simulink model "Backhoe_Arm_LS"  (R2013a)
settings: Solver=ode23t  StartTime=0.0  StopTime=30  MaxStep=0.01  RelTol=1e-3
PostLoadFcn:
  | warning off sm:compiler:state:UnsatisfiedDesiredTarget
  | warning off simscape:compiler:sli:init:SolverNotRecommended
  | warning off sm:sli:visualization:UnsupportedSimMode
  | warning off xPCTarget:sampleTime:sampleTimeInvariance
  | warning off sm:sli:setup:compile:LocalSolverNotSupported
model workspace (MAT data in the model file):
  cylinderGray = [0.6 0.6 0.6]
  darkOrange = [0.8 0.5 0]
  glassBlue = [0.2 0.2 1]
  gray = [0.3 0.3 0.3]
  orange = [0.8 0.65 0]
  pistonGray = [0.4 0.4 0.4]
  tireBlack = [0.1 0.1 0.1]
  wheelGray = [0.6 0.6 0.6]
  yellow = [0.8 0.8 0]
  rhoGlass = 2500
  rhoRubber = 1500
  rhoSteel = 7800
undefined symbols (not defined in the file or in its folder): BH_Param, sigbuilder_block, X, Y, Z
libraries: sm_lib x97, fl_lib x31, Backhoe_Lib x28, nesl_utility x21, sh_lib x9, xpclib x1
(part 2 of 4)

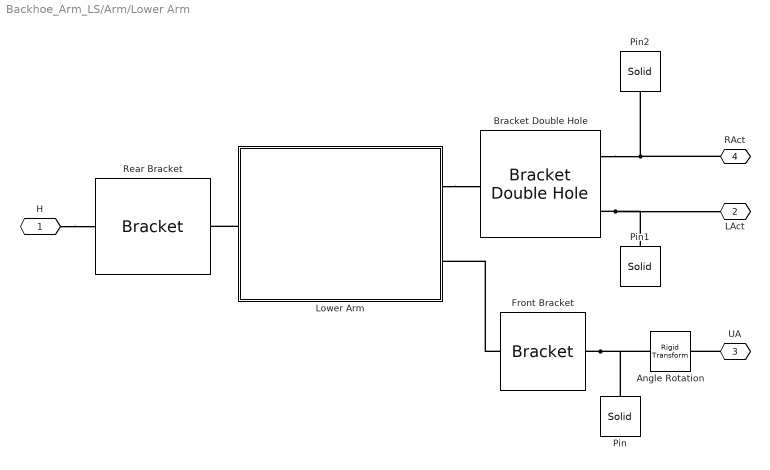
== system Backhoe_Arm_LS/Arm/Lower Arm  ==
  Angle Rotation : sm_lib/Frames and  Transforms/Rigid  Transform  TranslationMethod=None  TranslationLengthUnit=m  TranslationStandardAxis=+Z  TranslationStandardOffset=0  TranslationCartesianOffset=[0 0 0]  TranslationROffset=0  TranslationROffsetUnits=m  TranslationZOffset=0  TranslationZOffsetUnits=m  TranslationThetaOffset=0  TranslationThetaOffsetUnits=deg  RotationMethod=AlignedAxes  RotationAngleUnits=deg  RotationStandardAxis=+Z  RotationAngle=180  RotationArbitraryAxis=[0 0 1]  FollAlignAxisA=+Z  BaseAlignAxisA=+Z  FollAlignAxisB=+Y  BaseAlignAxisB=-Y  BlockFunction=simmechanics.library.frames_transforms.rigid_transform
  Bracket Double Hole : Backhoe_Lib/Bracket Double Hole  Hbracket=0.75  Wbracket=1.5  Tbracket=0.15  Dbracket=0.75  Hhole=0.5  Dhole=0.75  Rhole=0.075  Rfillet=0.375  Nc=25  bracketColor=orange  rho=rhoSteel
  Front Bracket : Backhoe_Lib/Bracket  Hbracket=0.65  Wbracket=0.5  Tbracket=0.225  Dbracket=0.45  Hhole=0.4  Rhole=0.075  circlePoints=25  bracketColor=darkOrange  rho=rhoSteel
  Lower Arm : Subsystem  mask(Lower Arm){Lbar=7, Wbar=0.8, Tbar=0.85, Lb=0.5, barFillet=0.1, numPoints=15, armColor=yellow, rho=rhoSteel}
      mask prompts: Lbar "Lbar [m]"; Wbar "Wbar [m]"; Tbar "Tbar [m]"; Lb "Lb [m]"; barFillet "Bar Fillet Radius [m]"; numPoints "Fillet Point Resolution"; armColor "Arm Color"; rho "Density [kg/m^3]"
      mask help:
      | Consists of the backhoe lower arm and three attachment brackets -- front, rear and upper
      |
      | Attachment Points are:
      | MA: Mounting Assembly attachment.
      | LH: Lower arm hydraulic actuator (piston Head).
      | UA: Upper arm attachment.
      | UC: Upper arm hydraulic actuator (Cylinder base).
      | All attachments are configured for Revolute joints.
      |
      | The length Lb corresponds to the lengths measured from the center of the bar to the center of the upper bracket.
      |
      | The front and rear brackets are automatically placed at the center of the end faces of the upper arm bar.
      |
      | Click on Help to view a schematic of the lower arm, its configurable dimension parameters and attachment points (in red).
      mask init:
      | barSection = [Tbar/2 Wbar/2;  ...
      |              -Tbar/2 Wbar/2;  ...
      |              -Tbar/2 -Wbar/2; ...
      |               Tbar/2 -Wbar/2];
      | barSection = Extr_Data_Round_Corners(barSection,1:4,barFillet,numPoints);
      mask Help: web('Backhoe_lowerarm.html');
      mask Display:
      | image(imread('Backhoe_Lowerarm_IMAGE.png'));
      | port_label('rconn',1,'RB');
      | port_label('lconn',2,'FB');;
      | port_label('lconn',1,'UB');
  Pin : sm_lib/Body Elements/Solid  InertiaType=CalculateFromGeometry  Mass=1  MassUnits=kg  CenterOfMass=[0 0 0]  CenterOfMassUnits=m  MomentsOfInertia=[1 1 1]  MomentsOfInertiaUnits=kg*m^2  ProductsOfInertia=[0 0 0]  ProductsOfInertiaUnits=kg*m^2  DensityBased=on  Density=rhoSteel  DensityUnits=kg/(m^3)  GraphicType=FromGeometry  MarkerShape=Sphere  MarkerSize=10  MarkerSizeUnits=m  GraphicVisPropType=SimpleVisualProperties  GraphicDiffuseColor=gray  GraphicSpecularColor=[0.5 0.5 0.5 1.0]  GraphicAmbientColor=[0.15 0.15 0.15 1.0]  GraphicEmissiveColor=[0.0 0.0 0.0 1.0]  GraphicShininess=75  GraphicOpacity=1.0  GeometryShape=Cylinder  RectangleSize=[1 1]  RectangleSizeUnits=m  BrickDimensions=[1 1 1]  BrickDimensionUnits=m  CylinderRadius=0.075  CylinderRadiusUnits=m  CylinderLength=0.8  CylinderLengthUnits=m  SphereRadius=1  SphereRadiusUnits=m  EllipsoidRadii=[1 1 1]  EllipsoidRadiiUnits=m  ExtrusionCrossSection=[1 1; -1 1; -1 -1; 1 -1]  ExtrusionCrossSectionUnits=m  ExtrusionLength=1  ExtrusionLengthUnits=m  PolygonNumSides=3  PolygonOuterRadius=1  PolygonOuterRadiusUnits=m  ExtGeomFileUnits=m  RevolutionCrossSection=[1 1; 1 -1; 2 -1; 2 1]  RevolutionCrossSectionUnits=m  RevolutionExtent=Full  RevolutionAngle=180  RevolutionAngleUnits=deg  BlockFunction=simmechanics.library.body_elements.solid
  Pin1 : sm_lib/Body Elements/Solid  InertiaType=CalculateFromGeometry  Mass=1  MassUnits=kg  CenterOfMass=[0 0 0]  CenterOfMassUnits=m  MomentsOfInertia=[1 1 1]  MomentsOfInertiaUnits=kg*m^2  ProductsOfInertia=[0 0 0]  ProductsOfInertiaUnits=kg*m^2  DensityBased=on  Density=rhoSteel  DensityUnits=kg/(m^3)  GraphicType=FromGeometry  MarkerShape=Sphere  MarkerSize=10  MarkerSizeUnits=m  GraphicVisPropType=SimpleVisualProperties  GraphicDiffuseColor=gray  GraphicSpecularColor=[0.5 0.5 0.5 1.0]  GraphicAmbientColor=[0.15 0.15 0.15 1.0]  GraphicEmissiveColor=[0.0 0.0 0.0 1.0]  GraphicShininess=75  GraphicOpacity=1.0  GeometryShape=Cylinder  RectangleSize=[1 1]  RectangleSizeUnits=m  BrickDimensions=[1 1 1]  BrickDimensionUnits=m  CylinderRadius=0.075  CylinderRadiusUnits=m  CylinderLength=0.8  CylinderLengthUnits=m  SphereRadius=1  SphereRadiusUnits=m  EllipsoidRadii=[1 1 1]  EllipsoidRadiiUnits=m  ExtrusionCrossSection=[1 1; -1 1; -1 -1; 1 -1]  ExtrusionCrossSectionUnits=m  ExtrusionLength=1  ExtrusionLengthUnits=m  PolygonNumSides=3  PolygonOuterRadius=1  PolygonOuterRadiusUnits=m  ExtGeomFileUnits=m  RevolutionCrossSection=[1 1; 1 -1; 2 -1; 2 1]  RevolutionCrossSectionUnits=m  RevolutionExtent=Full  RevolutionAngle=180  RevolutionAngleUnits=deg  BlockFunction=simmechanics.library.body_elements.solid
  Pin2 : sm_lib/Body Elements/Solid  InertiaType=CalculateFromGeometry  Mass=1  MassUnits=kg  CenterOfMass=[0 0 0]  CenterOfMassUnits=m  MomentsOfInertia=[1 1 1]  MomentsOfInertiaUnits=kg*m^2  ProductsOfInertia=[0 0 0]  ProductsOfInertiaUnits=kg*m^2  DensityBased=on  Density=rhoSteel  DensityUnits=kg/(m^3)  GraphicType=FromGeometry  MarkerShape=Sphere  MarkerSize=10  MarkerSizeUnits=m  GraphicVisPropType=SimpleVisualProperties  GraphicDiffuseColor=gray  GraphicSpecularColor=[0.5 0.5 0.5 1.0]  GraphicAmbientColor=[0.15 0.15 0.15 1.0]  GraphicEmissiveColor=[0.0 0.0 0.0 1.0]  GraphicShininess=75  GraphicOpacity=1.0  GeometryShape=Cylinder  RectangleSize=[1 1]  RectangleSizeUnits=m  BrickDimensions=[1 1 1]  BrickDimensionUnits=m  CylinderRadius=0.075  CylinderRadiusUnits=m  CylinderLength=0.8  CylinderLengthUnits=m  SphereRadius=1  SphereRadiusUnits=m  EllipsoidRadii=[1 1 1]  EllipsoidRadiiUnits=m  ExtrusionCrossSection=[1 1; -1 1; -1 -1; 1 -1]  ExtrusionCrossSectionUnits=m  ExtrusionLength=1  ExtrusionLengthUnits=m  PolygonNumSides=3  PolygonOuterRadius=1  PolygonOuterRadiusUnits=m  ExtGeomFileUnits=m  RevolutionCrossSection=[1 1; 1 -1; 2 -1; 2 1]  RevolutionCrossSectionUnits=m  RevolutionExtent=Full  RevolutionAngle=180  RevolutionAngleUnits=deg  BlockFunction=simmechanics.library.body_elements.solid
  Rear Bracket : Backhoe_Lib/Bracket  Hbracket=0.75  Wbracket=0.75  Tbracket=0.15  Dbracket=0.75  Hhole=0.5  Rhole=0.075  circlePoints=25  bracketColor=darkOrange  rho=rhoSteel
  H : PMIOPort  Port=1  Side=Left
  LAct : PMIOPort  Port=2  Side=Left
  UA : PMIOPort  Port=3  Side=Right
  RAct : PMIOPort  Port=4  Side=Right
  connections:
  H/RConn1 -- Rear Bracket/RConn1
  Lower Arm/RConn1 -- Rear Bracket/LConn1
  Front Bracket/RConn1 -- Pin/RConn1 -- Angle Rotation/LConn1
  Front Bracket/LConn1 -- Lower Arm/LConn2
  UA/RConn1 -- Angle Rotation/RConn1
  Lower Arm/LConn1 -- Bracket Double Hole/LConn1
  Bracket Double Hole/RConn2 -- LAct/RConn1 -- Pin1/RConn1
  Bracket Double Hole/RConn1 -- RAct/RConn1 -- Pin2/RConn1

== system Backhoe_Arm_LS/Arm/Measured ==
  Vector Concatenate : Concatenate  NumInputs=3
  Angles : Outport
  wires:
  [UA] -> Vector Concatenate/2
  Vector Concatenate/1 -> Angles/1
  [BuA] -> Vector Concatenate/1
  [LA] -> Vector Concatenate/3

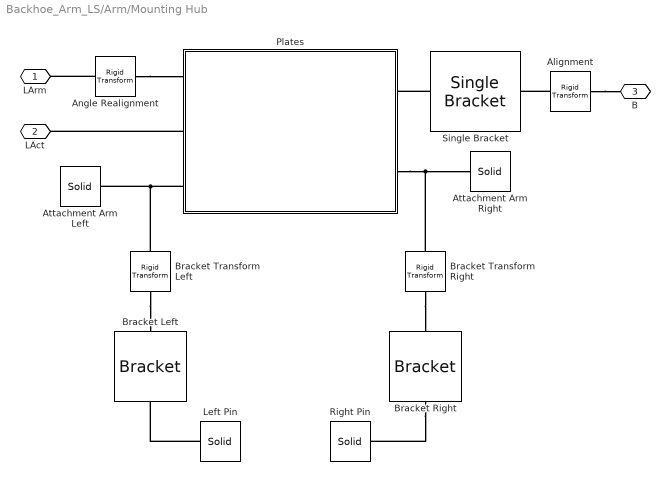
== system Backhoe_Arm_LS/Arm/Mounting Hub ==
  Alignment : sm_lib/Frames and  Transforms/Rigid  Transform  TranslationMethod=None  TranslationLengthUnit=m  TranslationStandardAxis=+Z  TranslationStandardOffset=0  TranslationCartesianOffset=[0 0 0]  TranslationROffset=0  TranslationROffsetUnits=m  TranslationZOffset=0  TranslationZOffsetUnits=m  TranslationThetaOffset=0  TranslationThetaOffsetUnits=deg  RotationMethod=StandardAxis  RotationAngleUnits=deg  RotationStandardAxis=+Y  RotationAngle=180  RotationArbitraryAxis=[0 0 1]  FollAlignAxisA=+X  BaseAlignAxisA=+X  FollAlignAxisB=+Y  BaseAlignAxisB=+Z  BlockFunction=simmechanics.library.frames_transforms.rigid_transform
  Angle Realignment : sm_lib/Frames and  Transforms/Rigid  Transform  TranslationMethod=None  TranslationLengthUnit=m  TranslationStandardAxis=+Z  TranslationStandardOffset=0.5  TranslationCartesianOffset=[ 0 0 0]  TranslationROffset=0  TranslationROffsetUnits=m  TranslationZOffset=0  TranslationZOffsetUnits=m  TranslationThetaOffset=0  TranslationThetaOffsetUnits=deg  RotationMethod=AlignedAxes  RotationAngleUnits=deg  RotationStandardAxis=-Z  RotationAngle=90  RotationArbitraryAxis=[0 0 1]  FollAlignAxisA=+Z  BaseAlignAxisA=+Z  FollAlignAxisB=+X  BaseAlignAxisB=-Y  BlockFunction=simmechanics.library.frames_transforms.rigid_transform
  Attachment Arm Left : sm_lib/Body Elements/Solid  InertiaType=CalculateFromGeometry  Mass=1  MassUnits=kg  CenterOfMass=[0 0 0]  CenterOfMassUnits=m  MomentsOfInertia=[1 1 1]  MomentsOfInertiaUnits=kg*m^2  ProductsOfInertia=[0 0 0]  ProductsOfInertiaUnits=kg*m^2  DensityBased=on  Density=rho  DensityUnits=kg/(m^3)  GraphicType=FromGeometry  MarkerShape=Sphere  MarkerSize=10  MarkerSizeUnits=m  GraphicVisPropType=SimpleVisualProperties  GraphicDiffuseColor=hubColor  GraphicSpecularColor=[0.5 0.5 0.5 1.0]  GraphicAmbientColor=[0.15 0.15 0.15 1.0]  GraphicEmissiveColor=[0.0 0.0 0.0 1.0]  GraphicShininess=75  GraphicOpacity=1.0  GeometryShape=Brick  RectangleSize=[1 1]  RectangleSizeUnits=m  BrickDimensions=[Warm Tarm (Larm-Warm)]  BrickDimensionUnits=m  CylinderRadius=1  CylinderRadiusUnits=m  CylinderLength=1  CylinderLengthUnits=m  SphereRadius=1  SphereRadiusUnits=m  EllipsoidRadii=[1 1 1]  EllipsoidRadiiUnits=m  ExtrusionCrossSection=plateSection  ExtrusionCrossSectionUnits=m  ExtrusionLength=Tplate  ExtrusionLengthUnits=m  PolygonNumSides=3  PolygonOuterRadius=1  PolygonOuterRadiusUnits=m  ExtGeomFileUnits=m  RevolutionCrossSection=[1 1; 1 -1; 2 -1; 2 1]  RevolutionCrossSectionUnits=m  RevolutionExtent=Full  RevolutionAngle=180  RevolutionAngleUnits=deg  BlockFunction=simmechanics.library.body_elements.solid
  Attachment Arm Right : sm_lib/Body Elements/Solid  InertiaType=CalculateFromGeometry  Mass=1  MassUnits=kg  CenterOfMass=[0 0 0]  CenterOfMassUnits=m  MomentsOfInertia=[1 1 1]  MomentsOfInertiaUnits=kg*m^2  ProductsOfInertia=[0 0 0]  ProductsOfInertiaUnits=kg*m^2  DensityBased=on  Density=rho  DensityUnits=kg/(m^3)  GraphicType=FromGeometry  MarkerShape=Sphere  MarkerSize=10  MarkerSizeUnits=m  GraphicVisPropType=SimpleVisualProperties  GraphicDiffuseColor=hubColor  GraphicSpecularColor=[0.5 0.5 0.5 1.0]  GraphicAmbientColor=[0.15 0.15 0.15 1.0]  GraphicEmissiveColor=[0.0 0.0 0.0 1.0]  GraphicShininess=75  GraphicOpacity=1.0  GeometryShape=Brick  RectangleSize=[1 1]  RectangleSizeUnits=m  BrickDimensions=[Warm Tarm (Larm-Warm)]  BrickDimensionUnits=m  CylinderRadius=1  CylinderRadiusUnits=m  CylinderLength=1  CylinderLengthUnits=m  SphereRadius=1  SphereRadiusUnits=m  EllipsoidRadii=[1 1 1]  EllipsoidRadiiUnits=m  ExtrusionCrossSection=plateSection  ExtrusionCrossSectionUnits=m  ExtrusionLength=Tplate  ExtrusionLengthUnits=m  PolygonNumSides=3  PolygonOuterRadius=1  PolygonOuterRadiusUnits=m  ExtGeomFileUnits=m  RevolutionCrossSection=[1 1; 1 -1; 2 -1; 2 1]  RevolutionCrossSectionUnits=m  RevolutionExtent=Full  RevolutionAngle=180  RevolutionAngleUnits=deg  BlockFunction=simmechanics.library.body_elements.solid
  Bracket Transform Left : sm_lib/Frames and  Transforms/Rigid  Transform  TranslationMethod=StandardAxis  TranslationLengthUnit=m  TranslationStandardAxis=+Z  TranslationStandardOffset=(Larm-Warm)/2  TranslationCartesianOffset=[0 0 0]  TranslationROffset=0  TranslationROffsetUnits=m  TranslationZOffset=0  TranslationZOffsetUnits=m  TranslationThetaOffset=0  TranslationThetaOffsetUnits=deg  RotationMethod=AlignedAxes  RotationAngleUnits=deg  RotationStandardAxis=+Y  RotationAngle=180  RotationArbitraryAxis=[0 0 1]  FollAlignAxisA=+Z  BaseAlignAxisA=+Z  FollAlignAxisB=+X  BaseAlignAxisB=+X  BlockFunction=simmechanics.library.frames_transforms.rigid_transform
  Bracket Transform Right : sm_lib/Frames and  Transforms/Rigid  Transform  TranslationMethod=StandardAxis  TranslationLengthUnit=m  TranslationStandardAxis=-Z  TranslationStandardOffset=(Larm-Warm)/2  TranslationCartesianOffset=[0 0 0]  TranslationROffset=0  TranslationROffsetUnits=m  TranslationZOffset=0  TranslationZOffsetUnits=m  TranslationThetaOffset=0  TranslationThetaOffsetUnits=deg  RotationMethod=AlignedAxes  RotationAngleUnits=deg  RotationStandardAxis=+Y  RotationAngle=180  RotationArbitraryAxis=[0 0 1]  FollAlignAxisA=+Z  BaseAlignAxisA=-Z  FollAlignAxisB=+Y  BaseAlignAxisB=+Y  BlockFunction=simmechanics.library.frames_transforms.rigid_transform
  Bracket Left : Backhoe_Lib/Bracket  Hbracket=Warm  Wbracket=Warm  Tbracket=Tab  Dbracket=Tarm  Hhole=Warm/2  Rhole=RH3  circlePoints=25  bracketColor=hubColor  rho=rho
  Bracket Right : Backhoe_Lib/Bracket  Hbracket=Warm  Wbracket=Warm  Tbracket=Tab  Dbracket=Tarm  Hhole=Warm/2  Rhole=RH3  circlePoints=25  bracketColor=hubColor  rho=rho
  Left Pin : sm_lib/Body Elements/Solid  InertiaType=CalculateFromGeometry  Mass=1  MassUnits=kg  CenterOfMass=[0 0 0]  CenterOfMassUnits=m  MomentsOfInertia=[1 1 1]  MomentsOfInertiaUnits=kg*m^2  ProductsOfInertia=[0 0 0]  ProductsOfInertiaUnits=kg*m^2  DensityBased=on  Density=rhoSteel  DensityUnits=kg/(m^3)  GraphicType=FromGeometry  MarkerShape=Sphere  MarkerSize=10  MarkerSizeUnits=m  GraphicVisPropType=SimpleVisualProperties  GraphicDiffuseColor=gray  GraphicSpecularColor=[0.5 0.5 0.5 1.0]  GraphicAmbientColor=[0.15 0.15 0.15 1.0]  GraphicEmissiveColor=[0.0 0.0 0.0 1.0]  GraphicShininess=75  GraphicOpacity=1.0  GeometryShape=Cylinder  RectangleSize=[1 1]  RectangleSizeUnits=m  BrickDimensions=[3 0.5 0.5]  BrickDimensionUnits=m  CylinderRadius=RH3  CylinderRadiusUnits=m  CylinderLength=Tarm*1.2  CylinderLengthUnits=m  SphereRadius=1  SphereRadiusUnits=m  EllipsoidRadii=[1 1 1]  EllipsoidRadiiUnits=m  ExtrusionCrossSection=[1 1; -1 1; -1 -1; 1 -1]  ExtrusionCrossSectionUnits=m  ExtrusionLength=1  ExtrusionLengthUnits=m  PolygonNumSides=3  PolygonOuterRadius=1  PolygonOuterRadiusUnits=m  ExtGeomFileUnits=m  RevolutionCrossSection=[1 1; 1 -1; 2 -1; 2 1]  RevolutionCrossSectionUnits=m  RevolutionExtent=Full  RevolutionAngle=180  RevolutionAngleUnits=deg  BlockFunction=simmechanics.library.body_elements.solid
  Plates : Subsystem
      mask Display:
      | image(imread('Backhoe_Mountingplates_IMAGE.png'));
      | port_label('lconn',1,'LA');
      | port_label('lconn',2,'LC');
      | port_label('lconn',3,'AAL');
      | port_label('rconn',1,'B');
      | port_label('rconn',2,'AAR');
  Right Pin : sm_lib/Body Elements/Solid  InertiaType=CalculateFromGeometry  Mass=1  MassUnits=kg  CenterOfMass=[0 0 0]  CenterOfMassUnits=m  MomentsOfInertia=[1 1 1]  MomentsOfInertiaUnits=kg*m^2  ProductsOfInertia=[0 0 0]  ProductsOfInertiaUnits=kg*m^2  DensityBased=on  Density=rhoSteel  DensityUnits=kg/(m^3)  GraphicType=FromGeometry  MarkerShape=Sphere  MarkerSize=10  MarkerSizeUnits=m  GraphicVisPropType=SimpleVisualProperties  GraphicDiffuseColor=gray  GraphicSpecularColor=[0.5 0.5 0.5 1.0]  GraphicAmbientColor=[0.15 0.15 0.15 1.0]  GraphicEmissiveColor=[0.0 0.0 0.0 1.0]  GraphicShininess=75  GraphicOpacity=1.0  GeometryShape=Cylinder  RectangleSize=[1 1]  RectangleSizeUnits=m  BrickDimensions=[3 0.5 0.5]  BrickDimensionUnits=m  CylinderRadius=RH3  CylinderRadiusUnits=m  CylinderLength=Tarm*1.2  CylinderLengthUnits=m  SphereRadius=1  SphereRadiusUnits=m  EllipsoidRadii=[1 1 1]  EllipsoidRadiiUnits=m  ExtrusionCrossSection=[1 1; -1 1; -1 -1; 1 -1]  ExtrusionCrossSectionUnits=m  ExtrusionLength=1  ExtrusionLengthUnits=m  PolygonNumSides=3  PolygonOuterRadius=1  PolygonOuterRadiusUnits=m  ExtGeomFileUnits=m  RevolutionCrossSection=[1 1; 1 -1; 2 -1; 2 1]  RevolutionCrossSectionUnits=m  RevolutionExtent=Full  RevolutionAngle=180  RevolutionAngleUnits=deg  BlockFunction=simmechanics.library.body_elements.solid
  Single Bracket : Backhoe_Lib/Single Bracket  Hbracket=Lbracket  Wbracket=Dplates-Tplate  Tbracket=Hright  Hhole=Hhole  Rhole=Rhole  Nc=25  bracketColor=orange  rho=rho
  LArm : PMIOPort  Port=1  Side=Right
  LAct : PMIOPort  Port=2  Side=Right
  B : PMIOPort  Port=3  Side=Left
  connections:
  Bracket Transform Right/RConn1 -- Bracket Right/LConn1
  Bracket Right/RConn1 -- Right Pin/RConn1
  Bracket Transform Right/LConn1 -- Plates/RConn2 -- Attachment Arm Right/RConn1
  Bracket Transform Left/RConn1 -- Bracket Left/LConn1
  Left Pin/RConn1 -- Bracket Left/RConn1
  Bracket Transform Left/LConn1 -- Plates/LConn3 -- Attachment Arm Left/RConn1
  Single Bracket/LConn1 -- Plates/RConn1
  Plates/LConn2 -- LAct/RConn1
  Alignment/LConn1 -- B/RConn1
  Alignment/RConn1 -- Single Bracket/RConn1
  Angle Realignment/LConn1 -- Plates/LConn1
  Angle Realignment/RConn1 -- LArm/RConn1

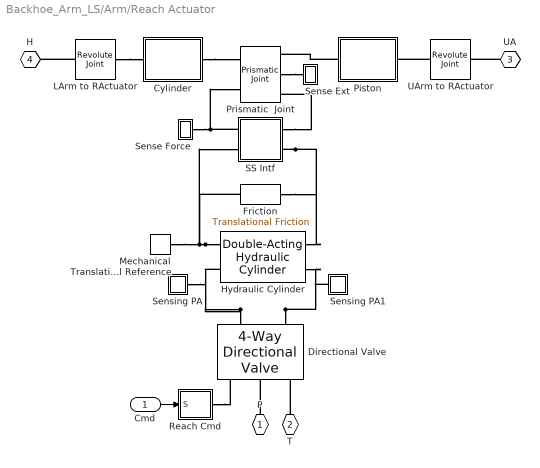
== system Backhoe_Arm_LS/Arm/Reach Actuator ==
  Cmd : Inport
  Cylinder : Subsystem
  Directional Valve : sh_lib/Valves/Directional Valves/4-Way Directional Valve  Tag=Factory Generic  mdl_type=1  area_max=hydr_valve_max_area mm^2  opening_max=hydr_valve_max_opening m  opening_tab="[  -0.002 0 0.005 0.015 ] m"  area_tab="[  1e-12 4e-12 1e-05 1.02e-05 ] m^2"  pressure_tab="[  -5e+06 -2e+06 2e+06 5e+06 ] Pa"  flow_rate_tab="[  -1e-12 -6e-14 6e+12 1e+11 ; -8e-08 -4e-08 4e+06 8e+06 ; -0.0025 -0.00103 0.001 0.0024 ; -0.00258 -0.001032 0.00106 0.00247 ; ] m^3/s"  interp_method=1  extrap_method=1  C_d=0.7  x_0_P_A=0 m  x_0_P_B=0 m  x_0_A_T=0 m  x_0_B_T=0 m  Re_cr=12  A_leak=1e-12 m^2  LocalVarLogging=[]
  Friction : fl_lib/Mechanical/Translational Elements/Translational Friction  brkwy_frc=friction_breakaway N  Col_frc=friction_coulomb N  visc_coef=friction_viscous N/(m/s)  trans_coef=10 s/m  vel_thr=1e-4 m/s  f_Log=off  v_Log=off  LocalVarNames=|f|v  LocalVarDescs=|f|v  LocalVarLogging=[0 0]
  Hydraulic Cylinder : sh_lib/Hydraulic Cylinders/Double-Acting Hydraulic Cylinder  Tag=Factory Generic  area_A=hydr_area m^2  area_B=hydr_area m^2  stroke=hydr_stroke m  init_pos=hydr_x0 m  dead_vol_A=hydr_deadvol m^3  dead_vol_B=hydr_deadvol m^3  init_pressure_A=hydr_PA0 Pa  init_pressure_B=hydr_PB0 Pa  k_sh=1.4  stiff=1e+06 N/m  D=150 N/(m/s)  or=2  LocalVarLogging=[]
  LArm to RActuator : sm_lib/Joints/Revolute Joint  SenseConstraintForceX=off  SenseConstraintForceY=off  SenseConstraintForceZ=off  SenseConstraintTorqueX=off  SenseConstraintTorqueY=off  SenseConstraintTorqueZ=off  ConstraintWrenchDir=FollowerOnBase  ConstraintWrenchFrame=BaseFrame  EquilibriumPosition=0  EquilibriumPositionUnits=deg  SpringStiffness=0  SpringStiffnessUnits=N*m/deg  DampingCoefficient=0  DampingCoefficientUnits=N*m/(deg/s)  ActuationMode=NoActuation  SensePosition=off  SenseVelocity=off  SenseAcceleration=off  SenseTorqueForce=off  PositionTargetValue=90  PositionTargetValueUnits=deg  PositionTargetSpecify=on  PositionTargetPriority=Low  VelocityTargetValue=0  VelocityTargetValueUnits=deg/s  VelocityTargetSpecify=off  VelocityTargetPriority=High  BlockFunction=simmechanics.library.joints.revolute_joint
  Mechanical Translational Reference : fl_lib/Mechanical/Translational Elements/Mechanical Translational Reference  Tag=Factory Generic  f_Log=off  LocalVarNames=|f  LocalVarDescs=|f  LocalVarLogging=[]
  Piston : Subsystem
  Prismatic  Joint : sm_lib/Joints/Prismatic  Joint  SenseConstraintForceX=off  SenseConstraintForceY=off  SenseConstraintForceZ=off  SenseConstraintTorqueX=off  SenseConstraintTorqueY=off  SenseConstraintTorqueZ=off  ConstraintWrenchDir=FollowerOnBase  ConstraintWrenchFrame=BaseFrame  EquilibriumPosition=0  EquilibriumPositionUnits=m  SpringStiffness=0  SpringStiffnessUnits=N/m  DampingCoefficient=0  DampingCoefficientUnits=N/(m/s)  ActuationMode=TorqueForceActuation  SensePosition=on  SenseVelocity=on  SenseAcceleration=off  SenseTorqueForce=off  PositionTargetValue=0  PositionTargetValueUnits=m  PositionTargetSpecify=off  PositionTargetPriority=Low  VelocityTargetValue=0  VelocityTargetValueUnits=m/s  VelocityTargetSpecify=off  VelocityTargetPriority=High  BlockFunction=simmechanics.library.joints.prismatic_joint
  Reach Cmd : Subsystem
  SS Intf : Subsystem
  Sense Ext : Subsystem
      mask Display: disp('S')
  Sense Force : Subsystem
      mask Display: disp('S')
  Sensing PA : Subsystem
      mask Display: disp('S')
  Sensing PA1 : Subsystem
      mask Display: disp('S')
  UArm to RActuator : sm_lib/Joints/Revolute Joint  SenseConstraintForceX=off  SenseConstraintForceY=off  SenseConstraintForceZ=off  SenseConstraintTorqueX=off  SenseConstraintTorqueY=off  SenseConstraintTorqueZ=off  ConstraintWrenchDir=FollowerOnBase  ConstraintWrenchFrame=BaseFrame  EquilibriumPosition=0  EquilibriumPositionUnits=deg  SpringStiffness=0  SpringStiffnessUnits=N*m/deg  DampingCoefficient=0  DampingCoefficientUnits=N*m/(deg/s)  ActuationMode=NoActuation  SensePosition=off  SenseVelocity=off  SenseAcceleration=off  SenseTorqueForce=off  PositionTargetValue=0  PositionTargetValueUnits=deg  PositionTargetSpecify=off  PositionTargetPriority=High  VelocityTargetValue=0  VelocityTargetValueUnits=deg/s  VelocityTargetSpecify=off  VelocityTargetPriority=High  BlockFunction=simmechanics.library.joints.revolute_joint
  P : PMIOPort  Port=1  Side=Left
  T : PMIOPort  Port=2  Side=Left
  UA : PMIOPort  Port=3  Side=Right
  H : PMIOPort  Port=4  Side=Right
  wires:
  Cmd/1 -> Reach Cmd/1(S)
  connections:
  Prismatic  Joint/RConn2 -- Sense Ext/LConn1
  Reach Cmd/RConn1 -- Directional Valve/RConn1
  T/RConn1 -- Directional Valve/RConn3
  P/RConn1 -- Directional Valve/RConn2
  LArm to RActuator/LConn1 -- H/RConn1
  Directional Valve/LConn2 -- Sensing PA1/LConn1 -- Hydraulic Cylinder/RConn2
  Hydraulic Cylinder/LConn1 -- SS Intf/RConn2 -- Friction/RConn1 -- Mechanical Translational Reference/LConn1
  Directional Valve/LConn1 -- Hydraulic Cylinder/LConn2 -- Sensing PA/LConn1
  SS Intf/LConn2 -- Hydraulic Cylinder/RConn1 -- Friction/LConn1
  Cylinder/LConn1 -- Prismatic  Joint/LConn1
  Piston/LConn1 -- Prismatic  Joint/RConn1
  SS Intf/LConn1 -- Prismatic  Joint/RConn3
  SS Intf/RConn1 -- Sense Force/RConn1 -- Prismatic  Joint/LConn2
  LArm to RActuator/RConn1 -- Cylinder/RConn1
  UA/RConn1 -- UArm to RActuator/RConn1
  UArm to RActuator/LConn1 -- Piston/RConn1

== system Backhoe_Arm_LS/Arm/Sensing AB ==
  PS-Simulink Converter Upper1 : nesl_utility/PS-Simulink Converter  PhysicalDomain=network_engine_domain  SubClassName=ps_output  LeftPortType=input  RightPortType=output  PseudoPeriodic=off  Frequencies=[]  Unit=deg  AffineConversion=off
  Conn1 : PMIOPort  Port=1  Side=Left
  tag scope: BuA=global
  wires:
  PS-Simulink Converter Upper1/1 -> [BuA]
  connections:
  PS-Simulink Converter Upper1/LConn1 -- Conn1/RConn1

== system Backhoe_Arm_LS/Arm/Sensing LAM ==
  PS-Simulink Converter Lower : nesl_utility/PS-Simulink Converter  PhysicalDomain=network_engine_domain  SubClassName=ps_output  LeftPortType=input  RightPortType=output  PseudoPeriodic=off  Frequencies=[]  Unit=deg  AffineConversion=off
  Conn1 : PMIOPort  Port=1  Side=Left
  tag scope: LA=global
  wires:
  PS-Simulink Converter Lower/1 -> [LA]
  connections:
  PS-Simulink Converter Lower/LConn1 -- Conn1/RConn1

== system Backhoe_Arm_LS/Arm/Sensing LAU ==
  PS-Simulink Converter Upper : nesl_utility/PS-Simulink Converter  PhysicalDomain=network_engine_domain  SubClassName=ps_output  LeftPortType=input  RightPortType=output  PseudoPeriodic=off  Frequencies=[]  Unit=deg  AffineConversion=off
  Conn1 : PMIOPort  Port=1  Side=Left
  tag scope: UA=global
  wires:
  PS-Simulink Converter Upper/1 -> [UA]
  connections:
  PS-Simulink Converter Upper/LConn1 -- Conn1/RConn1

== system Backhoe_Arm_LS/Arm/Sensing PA2 ==
  Hydraulic Flow Rate Sensor : fl_lib/Hydraulic/Hydraulic Sensors/Hydraulic Flow Rate Sensor  q_Log=off  p_Log=off  LocalVarNames=|q|p  LocalVarDescs=|q|p  LocalVarLogging=[0 0]
  Hydraulic Pressure Sensor : fl_lib/Hydraulic/Hydraulic Sensors/Hydraulic Pressure Sensor  q_Log=off  p_Log=off  LocalVarNames=|q|p  LocalVarDescs=|q|p  LocalVarLogging=[0 0]
  Hydraulic Reference1 : fl_lib/Hydraulic/Hydraulic Elements/Hydraulic Reference  q_Log=off  LocalVarNames=|q  LocalVarDescs=|q  LocalVarLogging=0
  PS-Simulink Converter1 : nesl_utility/PS-Simulink Converter  PhysicalDomain=network_engine_domain  SubClassName=ps_output  LeftPortType=input  RightPortType=output  PseudoPeriodic=off  Frequencies=[]  Unit=Pa  AffineConversion=off
  PS-Simulink Converter2 : nesl_utility/PS-Simulink Converter  PhysicalDomain=network_engine_domain  SubClassName=ps_output  LeftPortType=input  RightPortType=output  PseudoPeriodic=off  Frequencies=[]  Unit=lpm  AffineConversion=off
  A : PMIOPort  Port=1  Side=Left
  B : PMIOPort  Port=2  Side=Right
  tag scope: Pump_Flow=global, Pump_PP=global
  wires:
  PS-Simulink Converter1/1 -> [Pump_PP]
  PS-Simulink Converter2/1 -> [Pump_Flow]
  connections:
  Hydraulic Flow Rate Sensor/LConn1 -- A/RConn1 -- Hydraulic Pressure Sensor/LConn1
  Hydraulic Reference1/LConn1 -- Hydraulic Pressure Sensor/RConn1
  PS-Simulink Converter1/LConn1 -- Hydraulic Pressure Sensor/RConn2
  PS-Simulink Converter2/LConn1 -- Hydraulic Flow Rate Sensor/RConn1
  B/RConn1 -- Hydraulic Flow Rate Sensor/RConn2

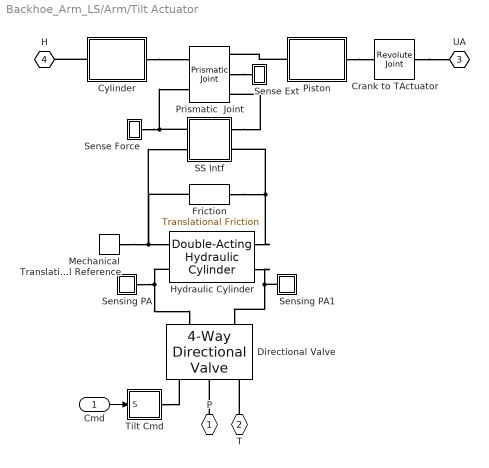
== system Backhoe_Arm_LS/Arm/Tilt Actuator ==
  Cmd : Inport
  Crank to TActuator : sm_lib/Joints/Revolute Joint  SenseConstraintForceX=off  SenseConstraintForceY=off  SenseConstraintForceZ=off  SenseConstraintTorqueX=off  SenseConstraintTorqueY=off  SenseConstraintTorqueZ=off  ConstraintWrenchDir=FollowerOnBase  ConstraintWrenchFrame=BaseFrame  EquilibriumPosition=0  EquilibriumPositionUnits=deg  SpringStiffness=0  SpringStiffnessUnits=N*m/deg  DampingCoefficient=0  DampingCoefficientUnits=N*m/(deg/s)  ActuationMode=NoActuation  SensePosition=off  SenseVelocity=off  SenseAcceleration=off  SenseTorqueForce=off  PositionTargetValue=0  PositionTargetValueUnits=deg  PositionTargetSpecify=off  PositionTargetPriority=High  VelocityTargetValue=0  VelocityTargetValueUnits=deg/s  VelocityTargetSpecify=off  VelocityTargetPriority=High  BlockFunction=simmechanics.library.joints.revolute_joint
  Cylinder : Subsystem
  Directional Valve : sh_lib/Valves/Directional Valves/4-Way Directional Valve  Tag=Factory Generic  mdl_type=1  area_max=hydr_valve_max_area mm^2  opening_max=hydr_valve_max_opening m  opening_tab="[  -0.002 0 0.005 0.015 ] m"  area_tab="[  1e-12 4e-12 1e-05 1.02e-05 ] m^2"  pressure_tab="[  -5e+06 -2e+06 2e+06 5e+06 ] Pa"  flow_rate_tab="[  -1e-12 -6e-14 6e+12 1e+11 ; -8e-08 -4e-08 4e+06 8e+06 ; -0.0025 -0.00103 0.001 0.0024 ; -0.00258 -0.001032 0.00106 0.00247 ; ] m^3/s"  interp_method=1  extrap_method=1  C_d=0.7  x_0_P_A=0 m  x_0_P_B=0 m  x_0_A_T=0 m  x_0_B_T=0 m  Re_cr=12  A_leak=1e-12 m^2  LocalVarLogging=[]
  Friction : fl_lib/Mechanical/Translational Elements/Translational Friction  brkwy_frc=friction_breakaway N  Col_frc=friction_coulomb N  visc_coef=friction_viscous N/(m/s)  trans_coef=10 s/m  vel_thr=1e-4 m/s  f_Log=off  v_Log=off  LocalVarNames=|f|v  LocalVarDescs=|f|v  LocalVarLogging=[0 0]
  Hydraulic Cylinder : sh_lib/Hydraulic Cylinders/Double-Acting Hydraulic Cylinder  Tag=Factory Generic  area_A=hydr_area m^2  area_B=hydr_area m^2  stroke=hydr_stroke m  init_pos=hydr_x0 m  dead_vol_A=hydr_deadvol m^3  dead_vol_B=hydr_deadvol m^3  init_pressure_A=hydr_PA0 Pa  init_pressure_B=hydr_PB0 Pa  k_sh=1.4  stiff=1e+06 N/m  D=150 N/(m/s)  or=2  LocalVarLogging=[]
  Mechanical Translational Reference : fl_lib/Mechanical/Translational Elements/Mechanical Translational Reference  Tag=Factory Generic  f_Log=off  LocalVarNames=|f  LocalVarDescs=|f  LocalVarLogging=[]
  Piston : Subsystem
  Prismatic  Joint : sm_lib/Joints/Prismatic  Joint  SenseConstraintForceX=off  SenseConstraintForceY=off  SenseConstraintForceZ=off  SenseConstraintTorqueX=off  SenseConstraintTorqueY=off  SenseConstraintTorqueZ=off  ConstraintWrenchDir=FollowerOnBase  ConstraintWrenchFrame=BaseFrame  EquilibriumPosition=0  EquilibriumPositionUnits=m  SpringStiffness=0  SpringStiffnessUnits=N/m  DampingCoefficient=0  DampingCoefficientUnits=N/(m/s)  ActuationMode=TorqueForceActuation  SensePosition=on  SenseVelocity=on  SenseAcceleration=off  SenseTorqueForce=off  PositionTargetValue=0  PositionTargetValueUnits=m  PositionTargetSpecify=off  PositionTargetPriority=Low  VelocityTargetValue=0  VelocityTargetValueUnits=m/s  VelocityTargetSpecify=off  VelocityTargetPriority=High  BlockFunction=simmechanics.library.joints.prismatic_joint
  SS Intf : Subsystem
  Sense Ext : Subsystem
      mask Display: disp('S')
  Sense Force : Subsystem
      mask Display: disp('S')
  Sensing PA : Subsystem
      mask Display: disp('S')
  Sensing PA1 : Subsystem
      mask Display: disp('S')
  Tilt Cmd : Subsystem
  P : PMIOPort  Port=1  Side=Left
  T : PMIOPort  Port=2  Side=Left
  UA : PMIOPort  Port=3  Side=Right
  H : PMIOPort  Port=4  Side=Right
  wires:
  Cmd/1 -> Tilt Cmd/1(S)
  connections:
  Crank to TActuator/RConn1 -- UA/RConn1
  SS Intf/RConn1 -- Sense Force/RConn1 -- Prismatic  Joint/LConn2
  SS Intf/LConn1 -- Prismatic  Joint/RConn3
  Piston/LConn1 -- Prismatic  Joint/RConn1
  Cylinder/LConn1 -- Prismatic  Joint/LConn1
  Friction/LConn1 -- Hydraulic Cylinder/RConn1 -- SS Intf/LConn2
  Sensing PA/LConn1 -- Hydraulic Cylinder/LConn2 -- Directional Valve/LConn1
  Mechanical Translational Reference/LConn1 -- Friction/RConn1 -- SS Intf/RConn2 -- Hydraulic Cylinder/LConn1
  Hydraulic Cylinder/RConn2 -- Sensing PA1/LConn1 -- Directional Valve/LConn2
  Cylinder/RConn1 -- H/RConn1
  P/RConn1 -- Directional Valve/RConn2
  T/RConn1 -- Directional Valve/RConn3
  Tilt Cmd/RConn1 -- Directional Valve/RConn1
  Prismatic  Joint/RConn2 -- Sense Ext/LConn1
  Piston/RConn1 -- Crank to TActuator/LConn1

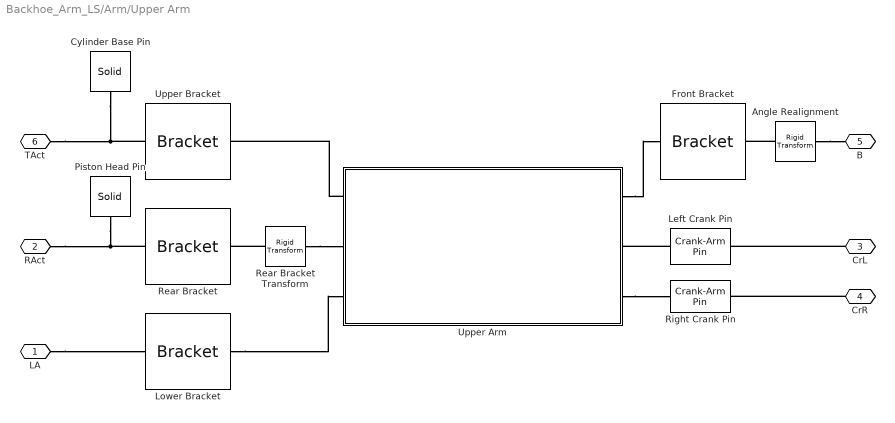
== system Backhoe_Arm_LS/Arm/Upper Arm ==
  Angle Realignment : sm_lib/Frames and  Transforms/Rigid  Transform  TranslationMethod=None  TranslationLengthUnit=m  TranslationStandardAxis=+Z  TranslationStandardOffset=0  TranslationCartesianOffset=[0 0 0]  TranslationROffset=0  TranslationROffsetUnits=m  TranslationZOffset=0  TranslationZOffsetUnits=m  TranslationThetaOffset=0  TranslationThetaOffsetUnits=deg  RotationMethod=AlignedAxes  RotationAngleUnits=deg  RotationStandardAxis=-Z  RotationAngle=90  RotationArbitraryAxis=[0 0 1]  FollAlignAxisA=+X  BaseAlignAxisA=-Y  FollAlignAxisB=+Z  BaseAlignAxisB=+Z  BlockFunction=simmechanics.library.frames_transforms.rigid_transform
  Cylinder Base Pin : sm_lib/Body Elements/Solid  InertiaType=CalculateFromGeometry  Mass=1  MassUnits=kg  CenterOfMass=[0 0 0]  CenterOfMassUnits=m  MomentsOfInertia=[1 1 1]  MomentsOfInertiaUnits=kg*m^2  ProductsOfInertia=[0 0 0]  ProductsOfInertiaUnits=kg*m^2  DensityBased=on  Density=rhoSteel  DensityUnits=kg/(m^3)  GraphicType=FromGeometry  MarkerShape=Sphere  MarkerSize=10  MarkerSizeUnits=m  GraphicVisPropType=SimpleVisualProperties  GraphicDiffuseColor=gray  GraphicSpecularColor=[0.5 0.5 0.5 1.0]  GraphicAmbientColor=[0.15 0.15 0.15 1.0]  GraphicEmissiveColor=[0.0 0.0 0.0 1.0]  GraphicShininess=75  GraphicOpacity=1.0  GeometryShape=Cylinder  RectangleSize=[1 1]  RectangleSizeUnits=m  BrickDimensions=[3 0.5 0.5]  BrickDimensionUnits=m  CylinderRadius=0.075  CylinderRadiusUnits=m  CylinderLength=0.8  CylinderLengthUnits=m  SphereRadius=1  SphereRadiusUnits=m  EllipsoidRadii=[1 1 1]  EllipsoidRadiiUnits=m  ExtrusionCrossSection=[1 1; -1 1; -1 -1; 1 -1]  ExtrusionCrossSectionUnits=m  ExtrusionLength=1  ExtrusionLengthUnits=m  PolygonNumSides=3  PolygonOuterRadius=1  PolygonOuterRadiusUnits=m  ExtGeomFileUnits=m  RevolutionCrossSection=[1 1; 1 -1; 2 -1; 2 1]  RevolutionCrossSectionUnits=m  RevolutionExtent=Full  RevolutionAngle=180  RevolutionAngleUnits=deg  BlockFunction=simmechanics.library.body_elements.solid
  Front Bracket : Backhoe_Lib/Bracket  Hbracket=0.65  Wbracket=0.5  Tbracket=0.15  Dbracket=0.625  Hhole=0.4  Rhole=0.075  circlePoints=25  bracketColor=orange  rho=rhoSteel
  Left Crank Pin : Backhoe_Lib/Crank-Arm Pin  R=0.075  L=0.25  T=0.2  color=gray  rho=rhoSteel
  Lower Bracket : Backhoe_Lib/Bracket  Hbracket=0.75  Wbracket=0.75  Tbracket=0.15  Dbracket=0.75  Hhole=0.5  Rhole=0.075  circlePoints=25  bracketColor=orange  rho=rhoSteel
  Piston Head Pin : sm_lib/Body Elements/Solid  InertiaType=CalculateFromGeometry  Mass=1  MassUnits=kg  CenterOfMass=[0 0 0]  CenterOfMassUnits=m  MomentsOfInertia=[1 1 1]  MomentsOfInertiaUnits=kg*m^2  ProductsOfInertia=[0 0 0]  ProductsOfInertiaUnits=kg*m^2  DensityBased=on  Density=rhoSteel  DensityUnits=kg/(m^3)  GraphicType=FromGeometry  MarkerShape=Sphere  MarkerSize=10  MarkerSizeUnits=m  GraphicVisPropType=SimpleVisualProperties  GraphicDiffuseColor=gray  GraphicSpecularColor=[0.5 0.5 0.5 1.0]  GraphicAmbientColor=[0.15 0.15 0.15 1.0]  GraphicEmissiveColor=[0.0 0.0 0.0 1.0]  GraphicShininess=75  GraphicOpacity=1.0  GeometryShape=Cylinder  RectangleSize=[1 1]  RectangleSizeUnits=m  BrickDimensions=[1 1 1]  BrickDimensionUnits=m  CylinderRadius=0.075  CylinderRadiusUnits=m  CylinderLength=0.8  CylinderLengthUnits=m  SphereRadius=1  SphereRadiusUnits=m  EllipsoidRadii=[1 1 1]  EllipsoidRadiiUnits=m  ExtrusionCrossSection=[1 1; -1 1; -1 -1; 1 -1]  ExtrusionCrossSectionUnits=m  ExtrusionLength=1  ExtrusionLengthUnits=m  PolygonNumSides=3  PolygonOuterRadius=1  PolygonOuterRadiusUnits=m  ExtGeomFileUnits=m  RevolutionCrossSection=[1 1; 1 -1; 2 -1; 2 1]  RevolutionCrossSectionUnits=m  RevolutionExtent=Full  RevolutionAngle=180  RevolutionAngleUnits=deg  BlockFunction=simmechanics.library.body_elements.solid
  Rear Bracket : Backhoe_Lib/Bracket  Hbracket=0.75  Wbracket=0.75  Tbracket=0.15  Dbracket=0.75  Hhole=0.5  Rhole=0.075  circlePoints=25  bracketColor=orange  rho=rhoSteel
  Rear Bracket Transform : sm_lib/Frames and  Transforms/Rigid  Transform  TranslationMethod=None  TranslationLengthUnit=m  TranslationStandardAxis=+Z  TranslationStandardOffset=0.5  TranslationCartesianOffset=[ 0 0 0]  TranslationROffset=0  TranslationROffsetUnits=m  TranslationZOffset=0  TranslationZOffsetUnits=m  TranslationThetaOffset=0  TranslationThetaOffsetUnits=deg  RotationMethod=AlignedAxes  RotationAngleUnits=deg  RotationStandardAxis=+X  RotationAngle=90  RotationArbitraryAxis=[0 0 1]  FollAlignAxisA=+Z  BaseAlignAxisA=+Z  FollAlignAxisB=+Y  BaseAlignAxisB=-Y  BlockFunction=simmechanics.library.frames_transforms.rigid_transform
  Right Crank Pin : Backhoe_Lib/Crank-Arm Pin  R=0.075  L=0.25  T=0.2  color=gray  rho=rhoSteel
  Upper Arm : Subsystem  mask(Upper Arm){Lbar=6, Wbar=0.8, Tbar=0.85, L1=1.5, L2=1.5, L3=2.5, barFillet=0.1, numPoints=15, Tcrank=0.2, armColor=yellow, rho=rhoSteel}
      mask prompts: Lbar "Lbar [m]"; Wbar "Wbar [m]"; Tbar "Tbar [m]"; L1 "L1 [m]"; L2 "L2 [m]"; L3 "L3 [m]"; barFillet "Bar Fillet Radius [m]"; numPoints "Fillet Point Resolution"; Tcrank "Crank Arm Thickness [m]"; armColor "Arm Color"; rho "Density [kg/m^3]"
      mask help:
      | Consists of the backhoe upper arm and four attachment brackets -- front, rear, upper and lower.
      |
      | Attachment points are:
      | B: Bucket attachment.
      | CL: Crank arm attachment (Left).
      | CR: Crank arm attachment (Right).
      | BC: Bucket hydraulic actuator (Cylinder base).
      | LA: Lower Arm attachment.
      | UH: Upper arm hydraulic actuator (piston Head).
      | All attachment points are configured for Revolute joints.
      |
      | The lengths L1, L2 and L3 correspond to lengths measured from the center of the bar, as follows:
      | L1: Upper Bracket
      | L2: Lower Bracket
      | L3: Crank Attachment Points
      | The front and rear brackets are automatically placed at the center of the end faces of the upper arm bar.
      |
      | Click on Help to view a schematic of the upper arm, its configurable dimension parameters and attachment points (in red).
      mask init: same as Backhoe_Arm_LS/Arm/Lower Arm /Lower Arm
      mask Help: web('Backhoe_Upperarm.html');
      mask Display:
      | image(imread('Backhoe_Upperbar_IMAGE.png'));
      | port_label('lconn',1,'CB');
      | port_label('lconn',2,'PH');
      | port_label('lconn',3,'LA');
      | port_label('rconn',1,'B');
      | port_label('rconn',2,'CL');
      | port_label('rconn',3,'CR');
  Upper Bracket : Backhoe_Lib/Bracket  Hbracket=0.75  Wbracket=0.75  Tbracket=0.15  Dbracket=0.75  Hhole=0.5  Rhole=0.075  circlePoints=25  bracketColor=orange  rho=rhoSteel
  LA : PMIOPort  Port=1  Side=Left
  RAct : PMIOPort  Port=2  Side=Left
  CrL : PMIOPort  Port=3  Side=Right
  CrR : PMIOPort  Port=4  Side=Right
  B : PMIOPort  Port=5  Side=Right
  TAct : PMIOPort  Port=6  Side=Right
  connections:
  Cylinder Base Pin/RConn1 -- Upper Bracket/RConn1 -- TAct/RConn1
  Piston Head Pin/RConn1 -- RAct/RConn1 -- Rear Bracket/RConn1
  Angle Realignment/LConn1 -- Front Bracket/RConn1
  LA/RConn1 -- Lower Bracket/RConn1
  CrL/RConn1 -- Left Crank Pin/LConn1
  CrR/RConn1 -- Right Crank Pin/LConn1
  Rear Bracket Transform/RConn1 -- Rear Bracket/LConn1
  Upper Arm/LConn1 -- Upper Bracket/LConn1
  Upper Arm/RConn1 -- Front Bracket/LConn1
  Upper Arm/RConn3 -- Right Crank Pin/RConn1
  Lower Bracket/LConn1 -- Upper Arm/LConn3
  Rear Bracket Transform/LConn1 -- Upper Arm/LConn2
  Left Crank Pin/RConn1 -- Upper Arm/RConn2
  Angle Realignment/RConn1 -- B/RConn1

== system Backhoe_Arm_LS/Arm/Bucket Assembly/Bucket ==
  Arm Revolute Rotation : sm_lib/Frames and  Transforms/Rigid  Transform  TranslationMethod=None  TranslationLengthUnit=m  TranslationStandardAxis=+X  TranslationStandardOffset=0  TranslationCartesianOffset=[0 0 0]  TranslationROffset=0  TranslationROffsetUnits=m  TranslationZOffset=0  TranslationZOffsetUnits=m  TranslationThetaOffset=0  TranslationThetaOffsetUnits=deg  RotationMethod=AlignedAxes  RotationAngleUnits=deg  RotationStandardAxis=-Y  RotationAngle=180  RotationArbitraryAxis=[0 0 1]  FollAlignAxisA=+Y  BaseAlignAxisA=+Y  FollAlignAxisB=+X  BaseAlignAxisB=-X  BlockFunction=simmechanics.library.frames_transforms.rigid_transform
  Attachment Frame : Subsystem
      mask Display:
      | image(imread('Backhoe_Attach_IMAGE.png'));
      | port_label('lconn',1,'B');
      | port_label('rconn',1,'CA');
      | port_label('rconn',2,'UA');
  Bucket : Subsystem
      mask Display:
      | image(imread('Backhoe_Bucketcase_IMAGE.png'));
      | port_label('rconn',1,'AF');
  Crank Revolute Rotation : sm_lib/Frames and  Transforms/Rigid  Transform  TranslationMethod=None  TranslationLengthUnit=m  TranslationStandardAxis=+X  TranslationStandardOffset=0  TranslationCartesianOffset=[0 0 0]  TranslationROffset=0  TranslationROffsetUnits=m  TranslationZOffset=0  TranslationZOffsetUnits=m  TranslationThetaOffset=0  TranslationThetaOffsetUnits=deg  RotationMethod=AlignedAxes  RotationAngleUnits=deg  RotationStandardAxis=-Y  RotationAngle=180  RotationArbitraryAxis=[0 0 1]  FollAlignAxisA=+Y  BaseAlignAxisA=+Y  FollAlignAxisB=+X  BaseAlignAxisB=-X  BlockFunction=simmechanics.library.frames_transforms.rigid_transform
  Crank Arm : PMIOPort  Port=1  Side=Right
  Upper Arm : PMIOPort  Port=2  Side=Right
  connections:
  Bucket/RConn1 -- Attachment Frame/LConn1
  Crank Revolute Rotation/LConn1 -- Attachment Frame/RConn1
  Arm Revolute Rotation/LConn1 -- Attachment Frame/RConn2
  Upper Arm/RConn1 -- Arm Revolute Rotation/RConn1
  Crank Arm/RConn1 -- Crank Revolute Rotation/RConn1

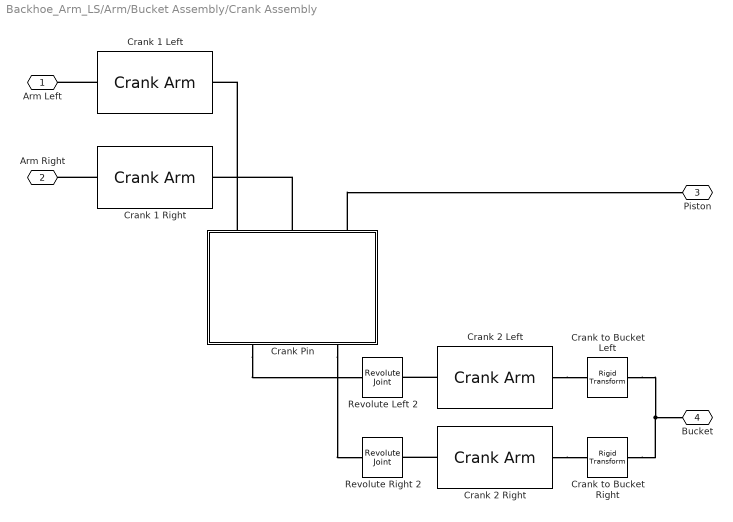
== system Backhoe_Arm_LS/Arm/Bucket Assembly/Crank Assembly ==
  Crank 1 Left : Backhoe_Lib/Crank Arm  L=LC1  W=WC1  T=TC1  D=DH1  R=Rpin  Nc=25  color=color1  rho=rho1
  Crank 1 Right : Backhoe_Lib/Crank Arm  L=LC1  W=WC1  T=TC1  D=DH1  R=Rpin  Nc=25  color=color1  rho=rho1
  Crank 2 Left : Backhoe_Lib/Crank Arm  L=LC2  W=WC2  T=TC2  D=DH2  R=Rpin  Nc=25  color=color2  rho=rho2
  Crank 2 Right : Backhoe_Lib/Crank Arm  L=LC2  W=WC2  T=TC2  D=DH2  R=Rpin  Nc=25  color=color2  rho=rho2
  Crank Pin : Subsystem
      mask Display:
      | image(repmat(imread('Backhoe_Crankpin_IMAGE.png'),[1 1 3]));
      | port_label('lconn',1,'C1L');
      | port_label('lconn',2,'C2L');
      | port_label('lconn',3,'PA');
      | port_label('rconn',1,'C2L');
      | port_label('rconn',2,'C2R');
  Crank to Bucket Right : sm_lib/Frames and  Transforms/Rigid  Transform  TranslationMethod=StandardAxis  TranslationLengthUnit=m  TranslationStandardAxis=+Z  TranslationStandardOffset=(DC2 - TC2)/2  TranslationCartesianOffset=[0 0 0]  TranslationROffset=0  TranslationROffsetUnits=m  TranslationZOffset=0  TranslationZOffsetUnits=m  TranslationThetaOffset=0  TranslationThetaOffsetUnits=deg  RotationMethod=None  RotationAngleUnits=deg  RotationStandardAxis=+Z  RotationAngle=0  RotationArbitraryAxis=[0 0 1]  FollAlignAxisA=+X  BaseAlignAxisA=+Y  FollAlignAxisB=+Y  BaseAlignAxisB=+Z  BlockFunction=simmechanics.library.frames_transforms.rigid_transform
  Crank to Bucket Left : sm_lib/Frames and  Transforms/Rigid  Transform  TranslationMethod=StandardAxis  TranslationLengthUnit=m  TranslationStandardAxis=-Z  TranslationStandardOffset=(DC2 - TC2)/2  TranslationCartesianOffset=[0 0 0]  TranslationROffset=0  TranslationROffsetUnits=m  TranslationZOffset=0  TranslationZOffsetUnits=m  TranslationThetaOffset=0  TranslationThetaOffsetUnits=deg  RotationMethod=None  RotationAngleUnits=deg  RotationStandardAxis=+Z  RotationAngle=0  RotationArbitraryAxis=[0 0 1]  FollAlignAxisA=+X  BaseAlignAxisA=+Y  FollAlignAxisB=+Y  BaseAlignAxisB=+Z  BlockFunction=simmechanics.library.frames_transforms.rigid_transform
  Revolute Left 2 : sm_lib/Joints/Revolute Joint  SenseConstraintForceX=off  SenseConstraintForceY=off  SenseConstraintForceZ=off  SenseConstraintTorqueX=off  SenseConstraintTorqueY=off  SenseConstraintTorqueZ=off  ConstraintWrenchDir=FollowerOnBase  ConstraintWrenchFrame=BaseFrame  EquilibriumPosition=0  EquilibriumPositionUnits=deg  SpringStiffness=0  SpringStiffnessUnits=N*m/deg  DampingCoefficient=0  DampingCoefficientUnits=N*m/(deg/s)  ActuationMode=NoActuation  SensePosition=off  SenseVelocity=off  SenseAcceleration=off  SenseTorqueForce=off  PositionTargetValue=-45  PositionTargetValueUnits=deg  PositionTargetSpecify=off  PositionTargetPriority=Low  VelocityTargetValue=0  VelocityTargetValueUnits=deg/s  VelocityTargetSpecify=off  VelocityTargetPriority=High  BlockFunction=simmechanics.library.joints.revolute_joint
  Revolute Right 2 : sm_lib/Joints/Revolute Joint  SenseConstraintForceX=off  SenseConstraintForceY=off  SenseConstraintForceZ=off  SenseConstraintTorqueX=off  SenseConstraintTorqueY=off  SenseConstraintTorqueZ=off  ConstraintWrenchDir=FollowerOnBase  ConstraintWrenchFrame=BaseFrame  EquilibriumPosition=0  EquilibriumPositionUnits=deg  SpringStiffness=0  SpringStiffnessUnits=N*m/deg  DampingCoefficient=0  DampingCoefficientUnits=N*m/(deg/s)  ActuationMode=NoActuation  SensePosition=off  SenseVelocity=off  SenseAcceleration=off  SenseTorqueForce=off  PositionTargetValue=0  PositionTargetValueUnits=deg  PositionTargetSpecify=off  PositionTargetPriority=High  VelocityTargetValue=0  VelocityTargetValueUnits=deg/s  VelocityTargetSpecify=off  VelocityTargetPriority=High  BlockFunction=simmechanics.library.joints.revolute_joint
  Arm Left : PMIOPort  Port=1  Side=Left
  Arm Right : PMIOPort  Port=2  Side=Left
  Piston : PMIOPort  Port=3  Side=Right
  Bucket : PMIOPort  Port=4  Side=Right
  connections:
  Crank Pin/RConn1 -- Revolute Left 2/LConn1
  Crank Pin/RConn2 -- Revolute Right 2/LConn1
  Crank 2 Left/LConn1 -- Revolute Left 2/RConn1
  Crank to Bucket Right/RConn1 -- Crank to Bucket Left/RConn1 -- Bucket/RConn1
  Crank Pin/LConn3 -- Piston/RConn1
  Crank 1 Left/RConn1 -- Arm Left/RConn1
  Crank 1 Right/RConn1 -- Arm Right/RConn1
  Crank Pin/LConn1 -- Crank 1 Left/LConn1
  Crank Pin/LConn2 -- Crank 1 Right/LConn1
  Crank 2 Right/LConn1 -- Revolute Right 2/RConn1
  Crank 2 Right/RConn1 -- Crank to Bucket Right/LConn1
  Crank 2 Left/RConn1 -- Crank to Bucket Left/LConn1

== system Backhoe_Arm_LS/Arm/Lift Actuator/Cylinder ==
  Base to Cylinder Transform : sm_lib/Frames and  Transforms/Rigid  Transform  TranslationMethod=StandardAxis  TranslationLengthUnit=m  TranslationStandardAxis=-Z  TranslationStandardOffset=(Lcyl/2)  TranslationCartesianOffset=[0 0 0]  TranslationROffset=0  TranslationROffsetUnits=m  TranslationZOffset=0  TranslationZOffsetUnits=m  TranslationThetaOffset=0  TranslationThetaOffsetUnits=deg  RotationMethod=AlignedAxes  RotationAngleUnits=deg  RotationStandardAxis=+X  RotationAngle=90  RotationArbitraryAxis=[0 0 1]  FollAlignAxisA=+X  BaseAlignAxisA=+X  FollAlignAxisB=+Z  BaseAlignAxisB=-Z  BlockFunction=simmechanics.library.frames_transforms.rigid_transform
  Cylinder : sm_lib/Body Elements/Solid  InertiaType=CalculateFromGeometry  Mass=1  MassUnits=kg  CenterOfMass=[0 0 0]  CenterOfMassUnits=m  MomentsOfInertia=[1 1 1]  MomentsOfInertiaUnits=kg*m^2  ProductsOfInertia=[0 0 0]  ProductsOfInertiaUnits=kg*m^2  DensityBased=on  Density=rhoCyl  DensityUnits=kg/(m^3)  GraphicType=FromGeometry  MarkerShape=Sphere  MarkerSize=10  MarkerSizeUnits=m  GraphicVisPropType=SimpleVisualProperties  GraphicDiffuseColor=cylColor  GraphicSpecularColor=[0.5 0.5 0.5 1.0]  GraphicAmbientColor=[0.15 0.15 0.15 1.0]  GraphicEmissiveColor=[0.0 0.0 0.0 1.0]  GraphicShininess=75  GraphicOpacity=1  GeometryShape=GeneralExtrusion  RectangleSize=[1 1]  RectangleSizeUnits=m  BrickDimensions=[3 0.5 0.5]  BrickDimensionUnits=m  CylinderRadius=Rcyl  CylinderRadiusUnits=m  CylinderLength=Lcyl  CylinderLengthUnits=m  SphereRadius=1  SphereRadiusUnits=m  EllipsoidRadii=[1 1 1]  EllipsoidRadiiUnits=m  ExtrusionCrossSection=cylSection  ExtrusionCrossSectionUnits=m  ExtrusionLength=Lcyl  ExtrusionLengthUnits=m  PolygonNumSides=3  PolygonOuterRadius=1  PolygonOuterRadiusUnits=m  ExtGeomFileUnits=m  RevolutionCrossSection=[1 1; 1 -1; 2 -1; 2 1]  RevolutionCrossSectionUnits=m  RevolutionExtent=Full  RevolutionAngle=180  RevolutionAngleUnits=deg  BlockFunction=simmechanics.library.body_elements.solid
  Single Bracket : Backhoe_Lib/Single Bracket  Hbracket=Lbase  Wbracket=Wbase  Tbracket=Wbase  Hhole=Lbase-(Wbase/2)  Rhole=Rbp  Nc=25  bracketColor=connColor  rho=rhoConn
  F : PMIOPort  Port=1  Side=Right
  B : PMIOPort  Port=2  Side=Left
  connections:
  Single Bracket/RConn1 -- F/RConn1
  Single Bracket/LConn1 -- Base to Cylinder Transform/RConn1
  Cylinder/RConn1 -- Base to Cylinder Transform/LConn1 -- B/RConn1

== system Backhoe_Arm_LS/Arm/Lift Actuator/Lift ==
  S : Inport
  Lift Cmd : Selector  InputPortWidth=3  IndexOptions=Index vector (dialog)  Indices=3  OutputSizes=1
  Simulink-PS Converter : nesl_utility/Simulink-PS Converter  PhysicalDomain=network_engine_domain  SubClassName=ps_input  LeftPortType=input  RightPortType=output  PseudoPeriodic=off  Frequencies=[]  NoiseDistribution=none  NoiseParameters=[]  Unit=1  AffineConversion=off  InputFiltering=off  SimscapeFilterOrder=1  InputFilterTimeConstant=.001  UdotUserProvided=0
  PS : PMIOPort  Port=1  Side=Right
  wires:
  Lift Cmd/1 -> Simulink-PS Converter/1
  S/1 -> Lift Cmd/1
  connections:
  Simulink-PS Converter/RConn1 -- PS/RConn1
